simulink model "p4"  (R2021b)
settings: Solver=VariableStepAuto  StartTime=0.0  StopTime=20  RelTol=1e-3
values from neighbouring files (symbols this model uses):
  A = [0 -0.378002311941 0 18.900115597 1 0 0 0 0 7.01473716863 0 -0.379715574203 ... (16 elements, 4x4)]    [Parameters.mat]
  B = [0 -0.0699290719413 0 3.49645359707]    [Parameters.mat]
  cx = [1 0 0 0]    [Parameters.mat]
  k1_fast = [94802.3767291 8696.07757469 3856.10279968 210.898086188]    [Parameters.mat]
  k1_slow = [59.3480374212 22.4783846411 34.1753242178 3.4774178969]    [Parameters.mat]
  k2_fast = -489885.003743    [Parameters.mat]
  k2_slow = -58.9710678899    [Parameters.mat]
libraries: simulink x2
settings Model: Creator=hp  LastModifiedBy=hp

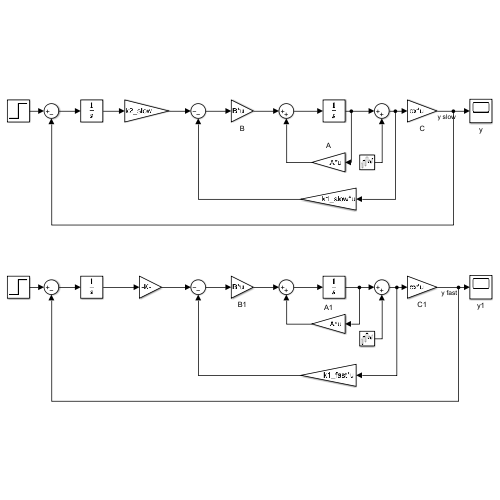
[thumbnail: Simulink's stored preview of the top-level diagram]
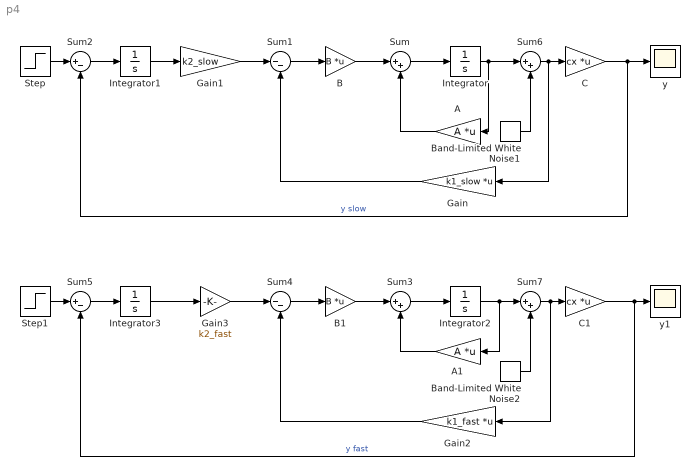
== system p4 ==
  A : Gain  Gain=A  Multiplication=Matrix(K*u)
  A1 : Gain  Gain=A  Multiplication=Matrix(K*u)
  B : Gain  Gain=B  Multiplication=Matrix(K*u)
  B1 : Gain  Gain=B  Multiplication=Matrix(K*u)
  Band-Limited White Noise1 : simulink/Sources/Band-Limited White Noise  Cov=[0.0002]  Ts=2  seed=[23341]
  Band-Limited White Noise2 : simulink/Sources/Band-Limited White Noise  Cov=[0.0002]  Ts=2  seed=[23341]
  C : Gain  Gain=cx  Multiplication=Matrix(K*u)
  C1 : Gain  Gain=cx  Multiplication=Matrix(K*u)
  Gain : Gain  Gain=k1_slow  Multiplication=Matrix(K*u)
  Gain1 : Gain  Gain=k2_slow
  Gain2 : Gain  Gain=k1_fast  Multiplication=Matrix(K*u)
  Gain3 : Gain  Gain=k2_fast
  Integrator : Integrator  InitialCondition=[0 0 0 0]
  Integrator1 : Integrator
  Integrator2 : Integrator  InitialCondition=[0 0 0 0]
  Integrator3 : Integrator
  Step : Step  Time=0  After=0.1  SampleTime=0
  Step1 : Step  Time=0  After=0.1  SampleTime=0
  Sum{,3,6..7} (4 alike) : Sum  Inputs=|++
  Sum1 : Sum  Inputs=|--
  Sum2 : Sum  Inputs=|+-
  Sum4 : Sum  Inputs=|--
  Sum5 : Sum  Inputs=|+-
  y : Scope
  y1 : Scope
  wires:
  A/1 -> Sum/2
  C/1 -> Sum2/2, y/1  "y slow"
  Sum/1 -> Integrator/1
  Gain/1 -> Sum1/2
  Sum1/1 -> B/1
  Gain1/1 -> Sum1/1
  Integrator1/1 -> Gain1/1
  Step/1 -> Sum2/1
  Sum2/1 -> Integrator1/1
  B/1 -> Sum/1
  Sum4/1 -> B1/1
  Gain2/1 -> Sum4/2
  C1/1 -> Sum5/2, y1/1  "y fast"
  B1/1 -> Sum3/1
  Sum3/1 -> Integrator2/1
  Integrator3/1 -> Gain3/1
  Gain3/1 -> Sum4/1
  Step1/1 -> Sum5/1
  A1/1 -> Sum3/2
  Sum5/1 -> Integrator3/1
  Integrator/1 -> A/1, Sum6/1
  Sum6/1 -> Gain/1, C/1
  Band-Limited White Noise1/1 -> Sum6/2
  Integrator2/1 -> A1/1, Sum7/1
  Band-Limited White Noise2/1 -> Sum7/2
  Sum7/1 -> Gain2/1, C1/1
